simulink model "sim_ES01"  (R2021b)
settings: Solver=VariableStepAuto  StartTime=0.0  StopTime=Ts  MaxStep=1e-02  RelTol=1e-3
values from neighbouring files (symbols this model uses):
  c = 2664    [DatiSospensione.m]    (also in Dati_Necessari.m; ES01_Comfort_4dof_stud.m = 0.00047; ES2_2DOF.m = C_values(count2); ES_2DOF_ANIM_TF.m = c_opt)
  choice2 = menu('Road profile h','Step signal h0 = 5cm','Sinewave','Chirp')    [ES_2DOF_ANIM_TF.m]
  h = 5/100    (= 0.05)    [Dati_Necessari.m]    (also in ES_2DOF_ANIM_TF.m)
  h0 = 2/100    (= 0.02)    [Dati_Necessari.m]    (also in ES01_Comfort_4dof_stud.m = 0.01; ES_2DOF_ANIM_TF.m)
  k = 35495    [DatiSospensione.m]    (also in Dati_Necessari.m = 99000; ES2_2DOF.m = 99000)
  lambda = 2    [Dati_Necessari.m]    (also in ES01_Comfort_4dof_stud.m = 2*pi*V./OM; ES_2DOF_ANIM_TF.m)
  m = ms+mu    (= 395)    [DatiSospensione.m]    (also in ES01_Comfort_4dof_stud.m = 1790)
  slope = h/0.01    (= 5)    [Dati_Necessari.m]    (also in ES_2DOF_ANIM_TF.m)
  T_sampling = 1/f_sampling    (= 0.001)    [Dati_Necessari.m]    (also in ES_2DOF_ANIM_TF.m)
  Ts = 4    [DatiSospensione.m]    (also in ES_2DOF_ANIM_TF.m = 100)
  v = 0    [Dati_Necessari.m]    (also in ES_2DOF_ANIM_TF.m = 36.1111111111)
  z0 = 0    [Dati_Necessari.m]    (also in ES_2DOF_ANIM_TF.m)
  zd0 = 0    [Dati_Necessari.m]    (also in ES_2DOF_ANIM_TF.m)
libraries: simulink x2
settings Model: Creator=Utente  LastModifiedBy=Utente
settings DataIOCC: ReturnWorkspaceOutputs=off

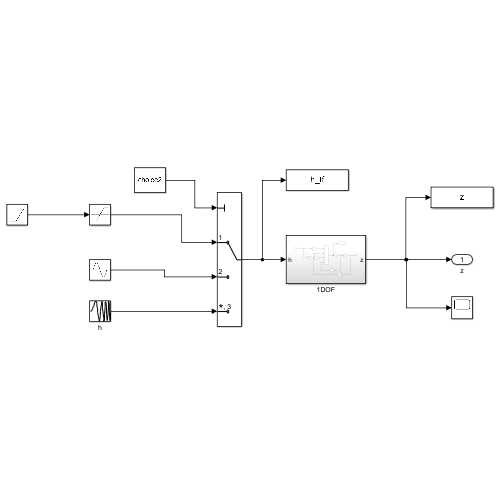
[thumbnail: Simulink's stored preview of the top-level diagram]
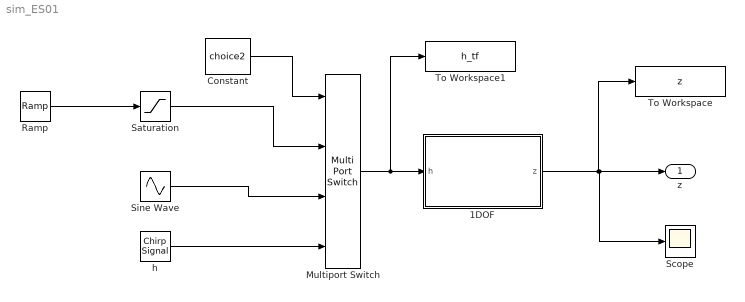
== system sim_ES01 ==
  1DOF : Subsystem
  Constant : Constant  Value=choice2
  Multiport Switch : MultiPortSwitch
  Ramp : simulink/Sources/Ramp  slope=slope  start=0.01  InitialOutput=0
  Saturation : Saturate  UpperLimit=h
  Scope : Scope
  Sine Wave : Sin  Amplitude=h0  Frequency=2*pi*v/lambda  SampleTime=0
  To Workspace : ToWorkspace  VariableName=z  SaveFormat=Timeseries  SampleTime=1/T_sampling
  To Workspace1 : ToWorkspace  VariableName=h_tf  SaveFormat=Timeseries  SampleTime=1/T_sampling
      settings: Decimation=decimation
  h : simulink/Sources/Chirp Signal  f1=w_in  T=Ts  f2=w_end
  z : Outport
  wires:
  1DOF/1(z) -> To Workspace/1, Scope/1, z/1
  Ramp/1 -> Saturation/1
  Constant/1 -> Multiport Switch/1
  Saturation/1 -> Multiport Switch/2
  Sine Wave/1 -> Multiport Switch/3
  Multiport Switch/1 -> To Workspace1/1, 1DOF/1(h)
  h/1 -> Multiport Switch/4

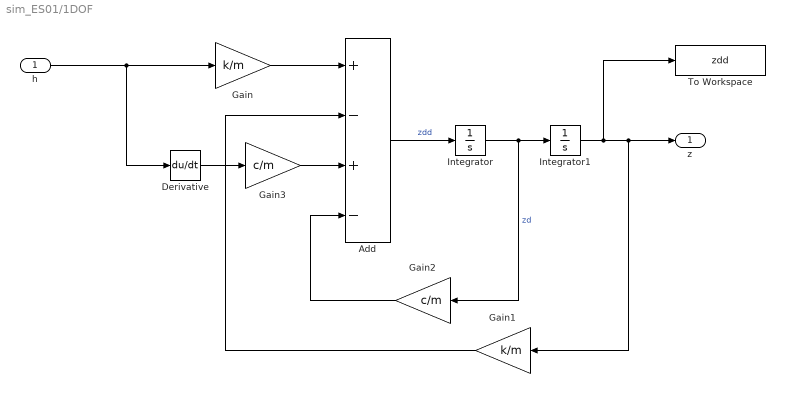
== system sim_ES01/1DOF ==
  h : Inport
  Add : Sum  Inputs=+-+-
  Derivative : Derivative
  Gain : Gain  Gain=k/m
  Gain1 : Gain  Gain=k/m
  Gain2 : Gain  Gain=c/m
  Gain3 : Gain  Gain=c/m
  Integrator : Integrator  InitialCondition=zd0
  Integrator1 : Integrator  InitialCondition=z0
  To Workspace : ToWorkspace  VariableName=zdd  SaveFormat=Timeseries  SampleTime=1/T_sampling
  z : Outport
  wires:
  Derivative/1 -> Gain3/1
  Add/1 -> Integrator/1  "zdd"
  h/1 -> Derivative/1, Gain/1
  Gain1/1 -> Add/2
  Integrator1/1 -> To Workspace/1, z/1, Gain1/1
  Gain/1 -> Add/1
  Gain3/1 -> Add/3
  Integrator/1 -> Gain2/1, Integrator1/1  "zd"
  Gain2/1 -> Add/4
